simulink model "battery_cell_model"  (R2022b)
settings: Solver=VariableStepAuto  StartTime=0.0  StopTime=t_final  MaxStep=0.1  RelTol=1e-3
values from neighbouring files (symbols this model uses):
  Battery_Model = 6    [OB_N_2_udds.mat]    (also in OB_N_3_(2).mat; OB_N_3_fs.mat = 5; OB_N_3_udds.mat; OB_N_4_udds.mat)
  c =     [OB_N_2_udds.mat]    (also in OB_N_3_(2).mat; OB_N_3_fs.mat; OB_N_3_udds.mat; OB_N_4_udds.mat)
  initial_n = [0.0224016218596 0.0224016218596 0.0224016218596 0.0224016218596 0.0224016218596 0.0224016218596 0.0224016218596 0.0224016218596 0.0224016218596 0.0224016218596 0.0224016218596 0.0224016218596 ... (32 elements, 1x32)]    [OB_N_2_udds.mat]    (also in OB_N_3_(2).mat = [0.0124453454776 0.0124453454776 0.0124453454776 0.012445345; OB_N_3_fs.mat = [0.0248906909552 0.0248906909552 0.0248906909552 0.024890690; OB_N_3_udds.mat; OB_N_4_udds.mat)
  initial_n_lm = [0.0224016218596 0.0224016218596 0.0224016218596 0.0224016218596 0.0224016218596 0.0224016218596 0.0224016218596 0.0224016218596 0.0224016218596 0.0224016218596 0.0224016218596 0.0224016218596 ... (49 elements, 1x49)]    [OB_N_2_udds.mat]    (also in OB_N_3_(2).mat = [0.0124453454776 0.0124453454776 0.0124453454776 0.012445345; OB_N_3_fs.mat = [0.0248906909552 0.0248906909552 0.0248906909552 0.024890690; OB_N_3_udds.mat; OB_N_4_udds.mat)
  initial_n_nm = [0.0224016218596 0.0224016218596 0.0224016218596 0.0224016218596 0.0224016218596 0.0224016218596 0.0224016218596 0.0224016218596 0.0224016218596 0.0224016218596 0.0224016218596 0.0224016218596 ... (49 elements, 1x49)]    [OB_N_2_udds.mat]    (also in OB_N_3_(2).mat = [0.0124453454776 0.0124453454776 0.0124453454776 0.012445345; OB_N_3_fs.mat = [0.0248906909552 0.0248906909552 0.0248906909552 0.024890690; OB_N_3_udds.mat; OB_N_4_udds.mat)
  initial_p = [0.002349018 0.002349018 0.002349018 0.002349018 0.002349018 0.002349018 0.002349018 0.002349018 0.002349018 0.002349018 0.002349018 0.002349018 ... (32 elements, 1x32)]    [OB_N_2_udds.mat]    (also in OB_N_3_(2).mat = [0.00900837 0.00900837 0.00900837 0.00900837 0.00900837 0.00; OB_N_3_fs.mat = [0.00068418 0.00068418 0.00068418 0.00068418 0.00068418 0.00; OB_N_3_udds.mat; OB_N_4_udds.mat)
  initial_p_lm = [0.002349018 0.002349018 0.002349018 0.002349018 0.002349018 0.002349018 0.002349018 0.002349018 0.002349018 0.002349018 0.002349018 0.002349018 ... (49 elements, 1x49)]    [OB_N_2_udds.mat]    (also in OB_N_3_(2).mat = [0.00900837 0.00900837 0.00900837 0.00900837 0.00900837 0.00; OB_N_3_fs.mat = [0.00068418 0.00068418 0.00068418 0.00068418 0.00068418 0.00; OB_N_3_udds.mat; OB_N_4_udds.mat)
  initial_p_nm = [0.002349018 0.002349018 0.002349018 0.002349018 0.002349018 0.002349018 0.002349018 0.002349018 0.002349018 0.002349018 0.002349018 0.002349018 ... (49 elements, 1x49)]    [OB_N_2_udds.mat]    (also in OB_N_3_(2).mat = [0.00900837 0.00900837 0.00900837 0.00900837 0.00900837 0.00; OB_N_3_fs.mat = [0.00068418 0.00068418 0.00068418 0.00068418 0.00068418 0.00; OB_N_3_udds.mat; OB_N_4_udds.mat)
  x_initial_n = [0.0224016218596 0]    [OB_N_2_udds.mat]    (also in OB_N_3_(2).mat = [0.0124453454776 0 0]; OB_N_3_fs.mat = [0.0248906909552 0 0]; OB_N_3_udds.mat = [0.0224016218596 0 0]; OB_N_4_udds.mat = [0.0224016218596 0 0 0])
  x_initial_n_pade = [-7348.24708226 0 0 0 0 0]    [OB_N_2_udds.mat]    (also in OB_N_3_(2).mat = [-4082.35949015 0 0 0 0 0]; OB_N_3_fs.mat = [-8164.71898029 0 0 0 0 0]; OB_N_3_udds.mat; OB_N_4_udds.mat)
  x_initial_n_pade_D = [-2.366529513 0 0 0]    [OB_N_2_udds.mat]    (also in OB_N_3_(2).mat = [-1.31473861834 0 0 0]; OB_N_3_fs.mat = [-0.000240313391395 0 0]; OB_N_3_udds.mat; OB_N_4_udds.mat)
  x_initial_p = [0.002349018 0]    [OB_N_2_udds.mat]    (also in OB_N_3_(2).mat = [0.00900837 0 0]; OB_N_3_fs.mat = [0.00068418 0 0]; OB_N_3_udds.mat = [0.002349018 0 0]; OB_N_4_udds.mat = [0.002349018 0 0 0])
  x_initial_p_pade = [1152.00829448 0 0 0 0 0]    [OB_N_2_udds.mat]    (also in OB_N_3_(2).mat = [4417.8958866 0 0 0 0 0]; OB_N_3_fs.mat = [335.53639645 0 0 0 0 0]; OB_N_3_udds.mat; OB_N_4_udds.mat)
  x_initial_p_pade_D = [1152.00829448 0 0 0]    [OB_N_2_udds.mat]    (also in OB_N_3_(2).mat = [4417.8958866 0 0 0]; OB_N_3_fs.mat = [335.53639645 0 0]; OB_N_3_udds.mat; OB_N_4_udds.mat)
settings Model: Creator=moonjihoon  LastModifiedBy=moonjihoon
settings SolverCC: AlgebraicLoopSolver=TrustRegion
settings DebuggingCC: UnconnectedInputMsg=warning  UnconnectedOutputMsg=warning  UnconnectedLineMsg=warning  SFMachineParentedDataDiag=warning
settings ModelReferenceCC: EnableRefExpFcnMdlSchedulingChecks=on
settings RTWCC: DLArmComputeVersion=19.05

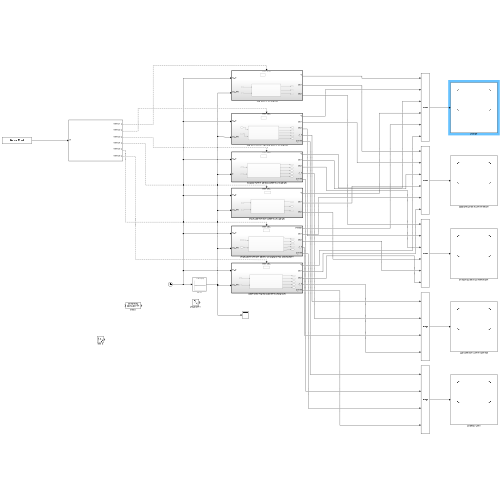
[thumbnail: Simulink's stored preview of the top-level diagram]
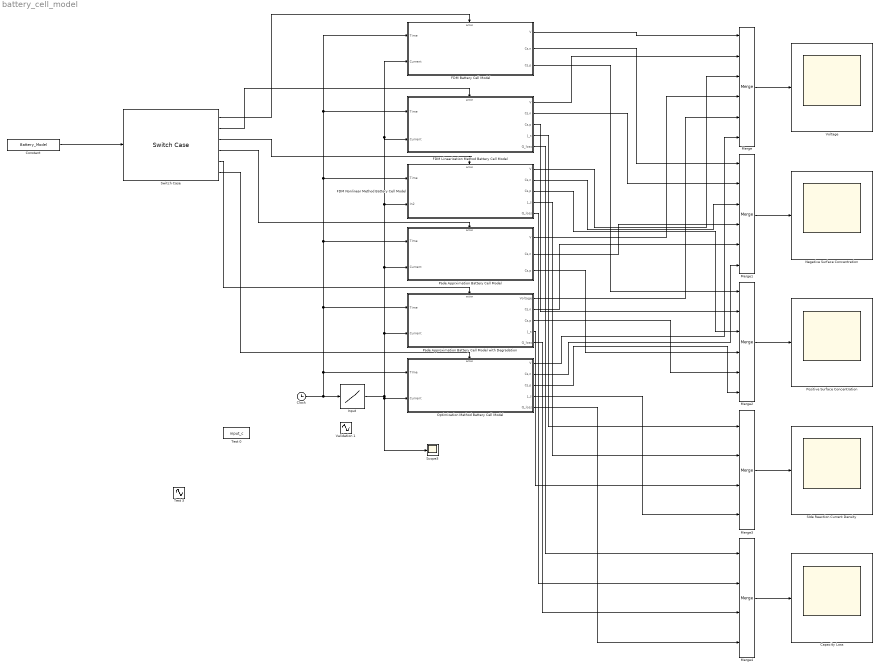
== system battery_cell_model ==
  Capacity Loss : Scope
  Clock : Clock
  Constant : Constant  Value=Battery_Model
  FDM Battery Cell Model : Subsystem  TreatAsAtomicUnit=on
  FDM Linearization Method Battery Cell Model : Subsystem  TreatAsAtomicUnit=on
  FDM Nonlinear Method Battery Cell Model : Subsystem  TreatAsAtomicUnit=on
  Input : Lookup_n-D  NumberOfTableDimensions=1  BreakpointsForDimension1=t  Table=u  InternalRulePriority=Speed  RndMeth=Simplest
  Merge : Merge  Inputs=6
  Merge1 : Merge  Inputs=6
  Merge2 : Merge  Inputs=6
  Merge3 : Merge  Inputs=4
  Merge4 : Merge  Inputs=4
  Negative Surface Concentration : Scope
  Optimization Method Battery Cell Model : Subsystem  TreatAsAtomicUnit=on
  Pade Approximation Battery Cell Model with Degradation : Subsystem  TreatAsAtomicUnit=on
  Pade Apprximation Battery Cell Model : Subsystem  TreatAsAtomicUnit=on
  Positive Surface Concentration : Scope
  SIde Reaction Current Density : Scope
  Scope3 : Scope
  Switch Case : SwitchCase  CaseConditions={1,2,3,4,5,6}  ShowDefaultCase=off
  Test 0 : MATLABFcn  MATLABFcn=input_c
  Test 3 : Sin  Amplitude=6  Frequency=0.03  Phase=3*pi/2  SampleTime=0
  Validation 1 : Sin  Amplitude=5  Frequency=0.02  SampleTime=0
  Voltage : Scope
  wires:
  Optimization Method Battery Cell Model/1(V) -> Merge/6
  Optimization Method Battery Cell Model/2(Cs,n) -> Merge1/6
  Optimization Method Battery Cell Model/3(Cs,p) -> Merge2/6
  FDM Battery Cell Model/2(Cs,n) -> Merge1/1
  FDM Battery Cell Model/3(Cs,p) -> Merge2/1
  FDM Battery Cell Model/1(V) -> Merge/1
  FDM Linearization Method Battery Cell Model/1(V) -> Merge/2
  FDM Linearization Method Battery Cell Model/2(Cs,n) -> Merge1/2
  FDM Linearization Method Battery Cell Model/3(Cs,p) -> Merge2/2
  FDM Linearization Method Battery Cell Model/4(J_s) -> Merge3/1
  FDM Nonlinear Method Battery Cell Model/1(V) -> Merge/3
  FDM Nonlinear Method Battery Cell Model/2(Cs,n) -> Merge1/3
  FDM Nonlinear Method Battery Cell Model/3(Cs,p) -> Merge2/3
  FDM Nonlinear Method Battery Cell Model/4(J_s) -> Merge3/2
  Pade Apprximation Battery Cell Model/1(V) -> Merge/4
  Pade Approximation Battery Cell Model with Degradation/3(Cs,p) -> Merge2/5
  Pade Approximation Battery Cell Model with Degradation/1(Voltage) -> Merge/5
  Pade Approximation Battery Cell Model with Degradation/2(Cs,n) -> Merge1/5
  Switch Case/1 -> FDM Battery Cell Model/Action
  Switch Case/2 -> FDM Linearization Method Battery Cell Model/Action
  Switch Case/3 -> FDM Nonlinear Method Battery Cell Model/Action
  Pade Apprximation Battery Cell Model/3(Cs,p) -> Merge2/4
  Pade Apprximation Battery Cell Model/2(Cs,n) -> Merge1/4
  Constant/1 -> Switch Case/1
  Switch Case/4 -> Pade Apprximation Battery Cell Model/Action
  Switch Case/5 -> Pade Approximation Battery Cell Model with Degradation/Action
  Switch Case/6 -> Optimization Method Battery Cell Model/Action
  Merge/1 -> Voltage/1
  Merge1/1 -> Negative Surface Concentration/1
  Merge2/1 -> Positive Surface Concentration/1
  Merge3/1 -> SIde Reaction Current Density/1
  FDM Linearization Method Battery Cell Model/5(Q_loss) -> Merge4/1
  Merge4/1 -> Capacity Loss/1
  FDM Nonlinear Method Battery Cell Model/5(Q_loss) -> Merge4/2
  Pade Approximation Battery Cell Model with Degradation/4(J_s) -> Merge3/3
  Pade Approximation Battery Cell Model with Degradation/5(Q_loss) -> Merge4/3
  Input/1 -> Optimization Method Battery Cell Model/2(Current), Scope3/1, Pade Apprximation Battery Cell Model/2(Current), FDM Nonlinear Method Battery Cell Model/2(In2), FDM Battery Cell Model/2(Current), FDM Linearization Method Battery Cell Model/2(Current), Pade Approximation Battery Cell Model with Degradation/2(Current)
  Clock/1 -> Input/1, Pade Apprximation Battery Cell Model/1(TIme), FDM Nonlinear Method Battery Cell Model/1(Time), FDM Battery Cell Model/1(Time), FDM Linearization Method Battery Cell Model/1(Time), Pade Approximation Battery Cell Model with Degradation/1(Time), Optimization Method Battery Cell Model/1(TIme)
  Optimization Method Battery Cell Model/4(J_s) -> Merge3/4
  Optimization Method Battery Cell Model/5(Q_loss) -> Merge4/4

== system battery_cell_model/FDM Battery Cell Model ==
  Time : Inport
  Current : Inport  Port=2
  Action Port : ActionPort  ActionPortLabel=case [ 1 ]:
  FDM Battery Cell Model : Subsystem
  V : Outport
  Cs,n : Outport  Port=2
  Cs,p : Outport  Port=3
  wires:
  Time/1 -> FDM Battery Cell Model/1(Time)
  Current/1 -> FDM Battery Cell Model/2(Current)
  FDM Battery Cell Model/1(V) -> V/1
  FDM Battery Cell Model/2(Cs,n) -> Cs,n/1
  FDM Battery Cell Model/3(Cs,p) -> Cs,p/1

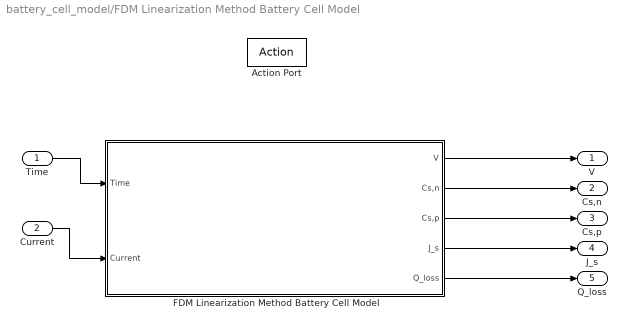
== system battery_cell_model/FDM Linearization Method Battery Cell Model ==
  Time : Inport
  Current : Inport  Port=2
  Action Port : ActionPort  ActionPortLabel=case [ 2 ]:
  FDM Linearization Method Battery Cell Model : Subsystem
  V : Outport
  Cs,n : Outport  Port=2
  Cs,p : Outport  Port=3
  J_s : Outport  Port=4
  Q_loss : Outport  Port=5
  wires:
  Time/1 -> FDM Linearization Method Battery Cell Model/1(Time)
  FDM Linearization Method Battery Cell Model/4(J_s) -> J_s/1
  Current/1 -> FDM Linearization Method Battery Cell Model/2(Current)
  FDM Linearization Method Battery Cell Model/1(V) -> V/1
  FDM Linearization Method Battery Cell Model/2(Cs,n) -> Cs,n/1
  FDM Linearization Method Battery Cell Model/3(Cs,p) -> Cs,p/1
  FDM Linearization Method Battery Cell Model/5(Q_loss) -> Q_loss/1

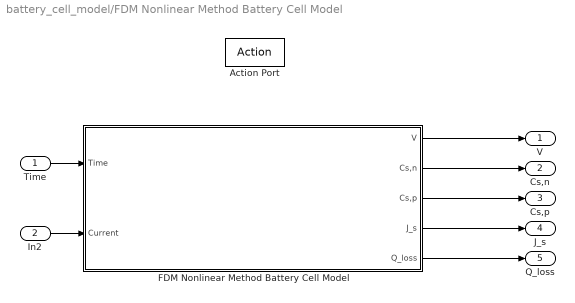
== system battery_cell_model/FDM Nonlinear Method Battery Cell Model ==
  Time : Inport
  In2 : Inport  Port=2
  Action Port : ActionPort  ActionPortLabel=case [ 3 ]:
  FDM Nonlinear Method Battery Cell Model : Subsystem
  V : Outport
  Cs,n : Outport  Port=2
  Cs,p : Outport  Port=3
  J_s : Outport  Port=4
  Q_loss : Outport  Port=5
  wires:
  In2/1 -> FDM Nonlinear Method Battery Cell Model/2(Current)
  Time/1 -> FDM Nonlinear Method Battery Cell Model/1(Time)
  FDM Nonlinear Method Battery Cell Model/1(V) -> V/1
  FDM Nonlinear Method Battery Cell Model/2(Cs,n) -> Cs,n/1
  FDM Nonlinear Method Battery Cell Model/3(Cs,p) -> Cs,p/1
  FDM Nonlinear Method Battery Cell Model/4(J_s) -> J_s/1
  FDM Nonlinear Method Battery Cell Model/5(Q_loss) -> Q_loss/1

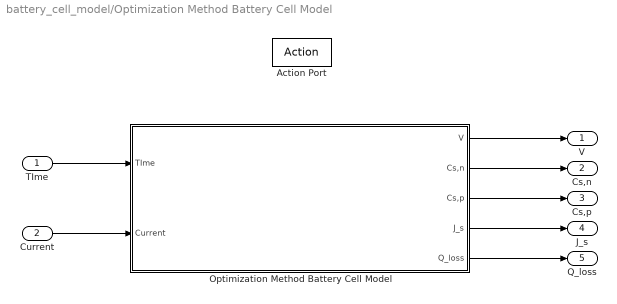
== system battery_cell_model/Optimization Method Battery Cell Model ==
  TIme : Inport
  Current : Inport  Port=2
  Action Port : ActionPort  ActionPortLabel=case [ 6 ]:
  Optimization Method Battery Cell Model : Subsystem
  V : Outport
  Cs,n : Outport  Port=2
  Cs,p : Outport  Port=3
  J_s : Outport  Port=4
  Q_loss : Outport  Port=5
  wires:
  Current/1 -> Optimization Method Battery Cell Model/2(Current)
  TIme/1 -> Optimization Method Battery Cell Model/1(TIme)
  Optimization Method Battery Cell Model/1(V) -> V/1
  Optimization Method Battery Cell Model/2(Cs,n) -> Cs,n/1
  Optimization Method Battery Cell Model/3(Cs,p) -> Cs,p/1
  Optimization Method Battery Cell Model/5(Q_loss) -> Q_loss/1
  Optimization Method Battery Cell Model/4(J_s) -> J_s/1

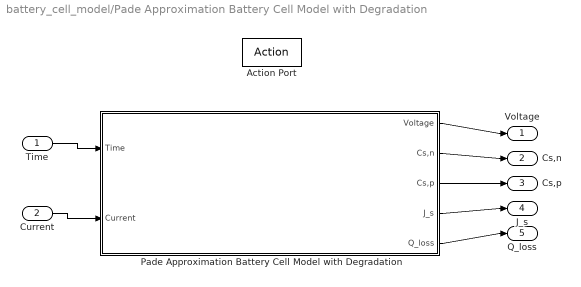
== system battery_cell_model/Pade Approximation Battery Cell Model with Degradation ==
  Time : Inport
  Current : Inport  Port=2
  Action Port : ActionPort  ActionPortLabel=case [ 5 ]:
  Pade Approximation Battery Cell Model with Degradation : Subsystem
  Voltage : Outport
  Cs,n : Outport  Port=2
  Cs,p : Outport  Port=3
  J_s : Outport  Port=4
  Q_loss : Outport  Port=5
  wires:
  Current/1 -> Pade Approximation Battery Cell Model with Degradation/2(Current)
  Time/1 -> Pade Approximation Battery Cell Model with Degradation/1(Time)
  Pade Approximation Battery Cell Model with Degradation/3(Cs,p) -> Cs,p/1
  Pade Approximation Battery Cell Model with Degradation/2(Cs,n) -> Cs,n/1
  Pade Approximation Battery Cell Model with Degradation/1(Voltage) -> Voltage/1
  Pade Approximation Battery Cell Model with Degradation/4(J_s) -> J_s/1
  Pade Approximation Battery Cell Model with Degradation/5(Q_loss) -> Q_loss/1

== system battery_cell_model/Pade Apprximation Battery Cell Model ==
  TIme : Inport
  Current : Inport  Port=2
  Action Port : ActionPort  ActionPortLabel=case [ 4 ]:
  Pade Apprximation Battery Cell Model : Subsystem
  V : Outport
  Cs,n : Outport  Port=2
  Cs,p : Outport  Port=3
  wires:
  Pade Apprximation Battery Cell Model/1(V) -> V/1
  Pade Apprximation Battery Cell Model/2(Cs,n) -> Cs,n/1
  Pade Apprximation Battery Cell Model/3(Cs,p) -> Cs,p/1
  Current/1 -> Pade Apprximation Battery Cell Model/2(Current)
  TIme/1 -> Pade Apprximation Battery Cell Model/1(TIme)

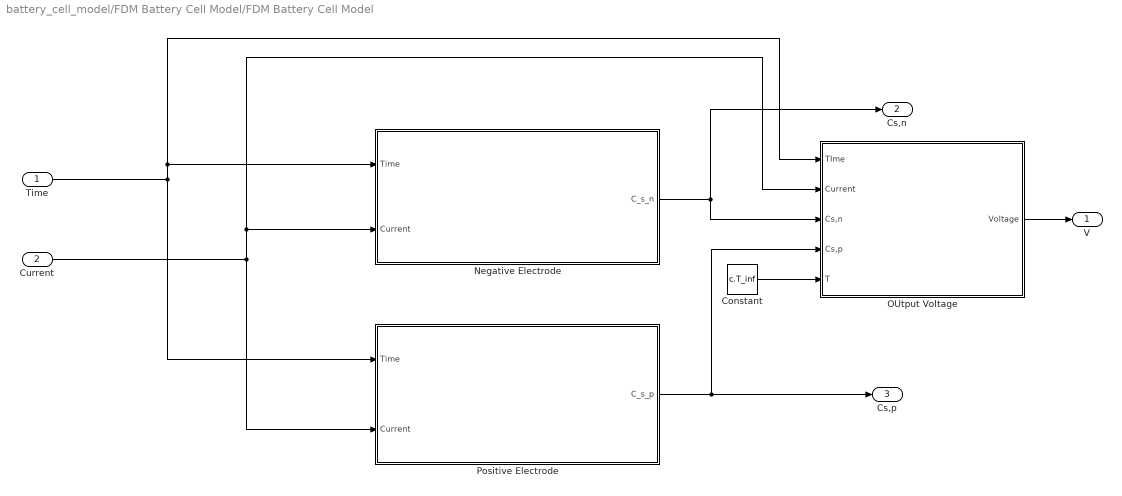
== system battery_cell_model/FDM Battery Cell Model/FDM Battery Cell Model ==
  Time : Inport
  Current : Inport  Port=2
  Constant : Constant  Value=c.T_inf
  Negative Electrode : Subsystem
  OUtput Voltage : Subsystem
  Positive Electrode : Subsystem
  V : Outport
  Cs,n : Outport  Port=2
  Cs,p : Outport  Port=3
  wires:
  Time/1 -> Negative Electrode/1(Time), OUtput Voltage/1(TIme), Positive Electrode/1(Time)
  Current/1 -> OUtput Voltage/2(Current), Negative Electrode/2(Current), Positive Electrode/2(Current)
  Constant/1 -> OUtput Voltage/5(T)
  OUtput Voltage/1(Voltage) -> V/1
  Negative Electrode/1(C_s_n) -> Cs,n/1, OUtput Voltage/3(Cs,n)
  Positive Electrode/1(C_s_p) -> OUtput Voltage/4(Cs,p), Cs,p/1

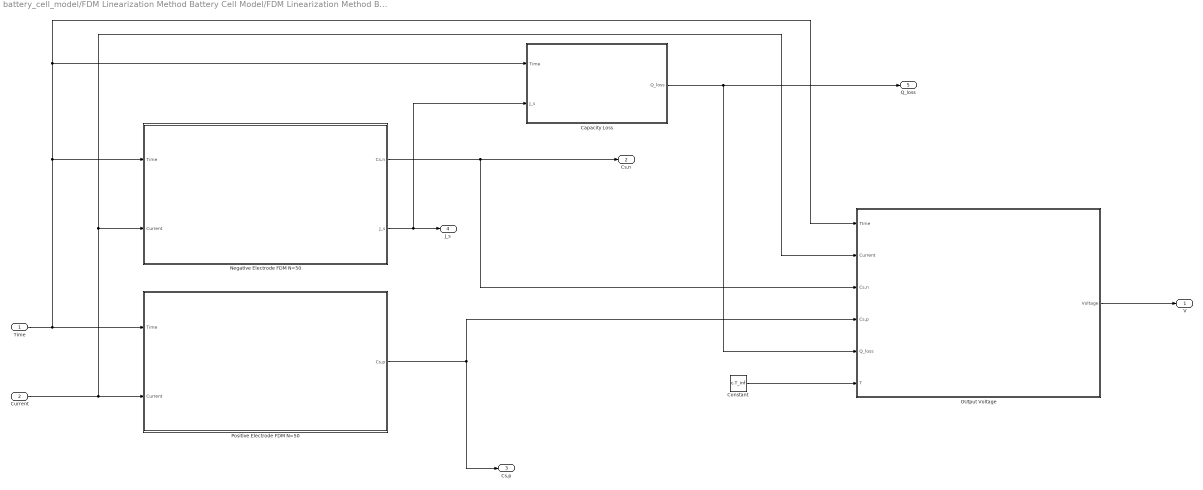
== system battery_cell_model/FDM Linearization Method Battery Cell Model/FDM Linearization Method Battery Cell Model ==
  Time : Inport
  Current : Inport  Port=2
  Capacity Loss : Subsystem
  Constant : Constant  Value=c.T_inf
  Negative Electrode FDM N=50 : Subsystem
  OUtput Voltage : Subsystem
  Positive Electrode FDM N=50 : Subsystem
  V : Outport
  Cs,n : Outport  Port=2
  Cs,p : Outport  Port=3
  J_s : Outport  Port=4
  Q_loss : Outport  Port=5
  wires:
  Constant/1 -> OUtput Voltage/6(T)
  Positive Electrode FDM N=50/1(Cs,p) -> Cs,p/1, OUtput Voltage/4(Cs,p)
  OUtput Voltage/1(Voltage) -> V/1
  Current/1 -> Negative Electrode FDM N=50/2(Current), OUtput Voltage/2(Current), Positive Electrode FDM N=50/2(Current)
  Negative Electrode FDM N=50/2(J_s) -> Capacity Loss/2(J_s), J_s/1
  Negative Electrode FDM N=50/1(Cs,n) -> OUtput Voltage/3(Cs,n), Cs,n/1
  Time/1 -> Capacity Loss/1(Time), OUtput Voltage/1(TIme), Negative Electrode FDM N=50/1(Time), Positive Electrode FDM N=50/1(Time)
  Capacity Loss/1(Q_loss) -> Q_loss/1, OUtput Voltage/5(Q_loss)

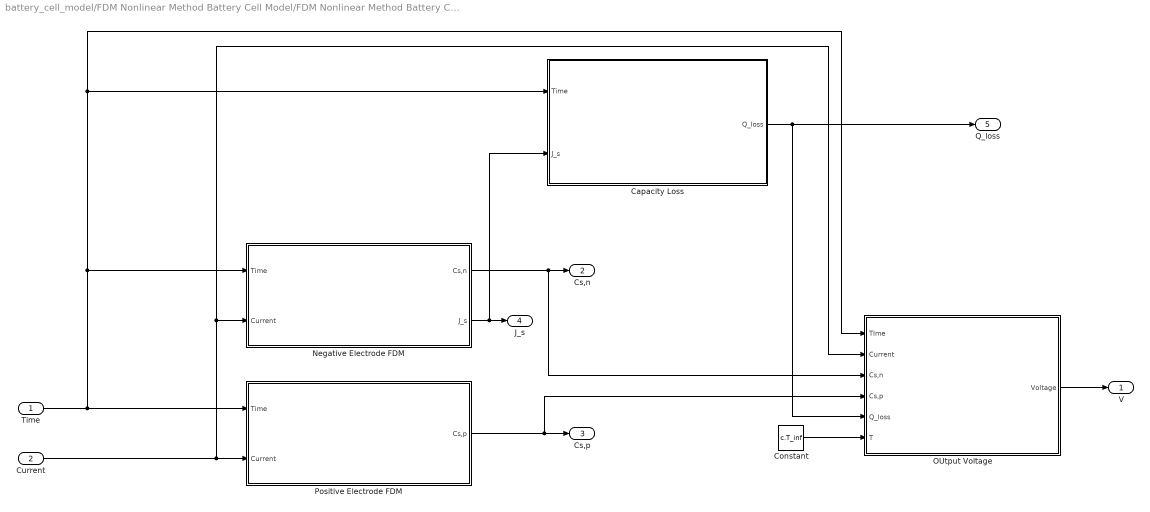
== system battery_cell_model/FDM Nonlinear Method Battery Cell Model/FDM Nonlinear Method Battery Cell Model ==
  Time : Inport
  Current : Inport  Port=2
  Capacity Loss : Subsystem
  Constant : Constant  Value=c.T_inf
  Negative Electrode FDM : Subsystem
  OUtput Voltage : Subsystem
  Positive Electrode FDM : Subsystem
  V : Outport
  Cs,n : Outport  Port=2
  Cs,p : Outport  Port=3
  J_s : Outport  Port=4
  Q_loss : Outport  Port=5
  wires:
  Negative Electrode FDM/2(J_s) -> Capacity Loss/2(J_s), J_s/1
  OUtput Voltage/1(Voltage) -> V/1
  Time/1 -> Negative Electrode FDM/1(Time), Capacity Loss/1(Time), OUtput Voltage/1(TIme), Positive Electrode FDM/1(Time)
  Positive Electrode FDM/1(Cs,p) -> OUtput Voltage/4(Cs,p), Cs,p/1
  Current/1 -> Negative Electrode FDM/2(Current), OUtput Voltage/2(Current), Positive Electrode FDM/2(Current)
  Constant/1 -> OUtput Voltage/6(T)
  Negative Electrode FDM/1(Cs,n) -> OUtput Voltage/3(Cs,n), Cs,n/1
  Capacity Loss/1(Q_loss) -> Q_loss/1, OUtput Voltage/5(Q_loss)

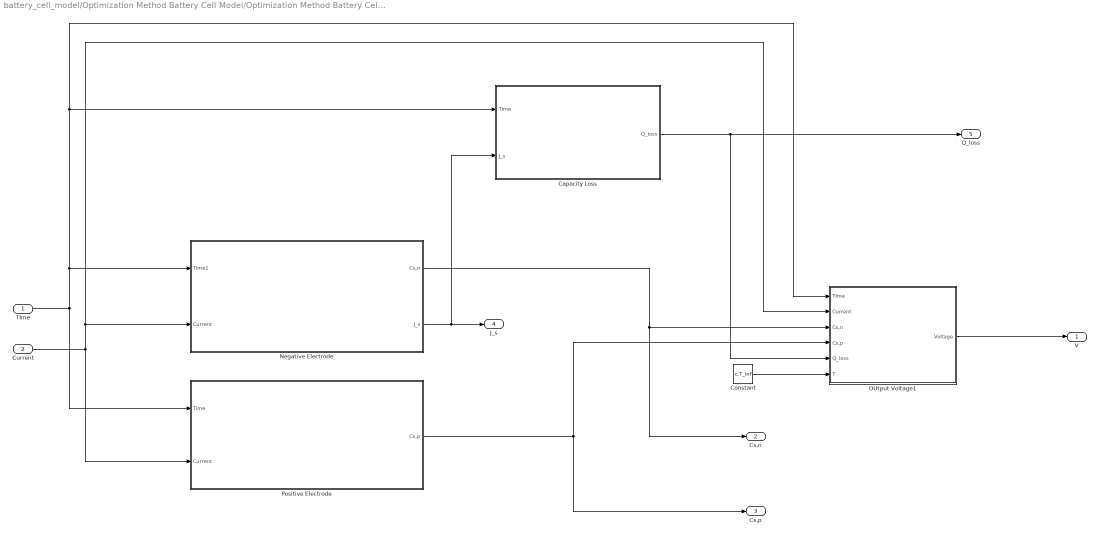
== system battery_cell_model/Optimization Method Battery Cell Model/Optimization Method Battery Cell Model ==
  TIme : Inport
  Current : Inport  Port=2
  Capacity Loss : Subsystem
  Constant : Constant  Value=c.T_inf
  Negative Electrode : Subsystem
  OUtput Voltage1 : Subsystem
  Positive Electrode : Subsystem
  V : Outport
  Cs,n : Outport  Port=2
  Cs,p : Outport  Port=3
  J_s : Outport  Port=4
  Q_loss : Outport  Port=5
  wires:
  Current/1 -> OUtput Voltage1/2(Current), Negative Electrode/2(Current), Positive Electrode/2(Current)
  TIme/1 -> Positive Electrode/1(Time), Capacity Loss/1(Time), OUtput Voltage1/1(TIme), Negative Electrode/1(Time1)
  OUtput Voltage1/1(Voltage) -> V/1
  Negative Electrode/1(Cs,n) -> Cs,n/1, OUtput Voltage1/3(Cs,n)
  Positive Electrode/1(Cs,p) -> Cs,p/1, OUtput Voltage1/4(Cs,p)
  Negative Electrode/2(J_s) -> Capacity Loss/2(J_s), J_s/1
  Capacity Loss/1(Q_loss) -> OUtput Voltage1/5(Q_loss), Q_loss/1
  Constant/1 -> OUtput Voltage1/6(T)

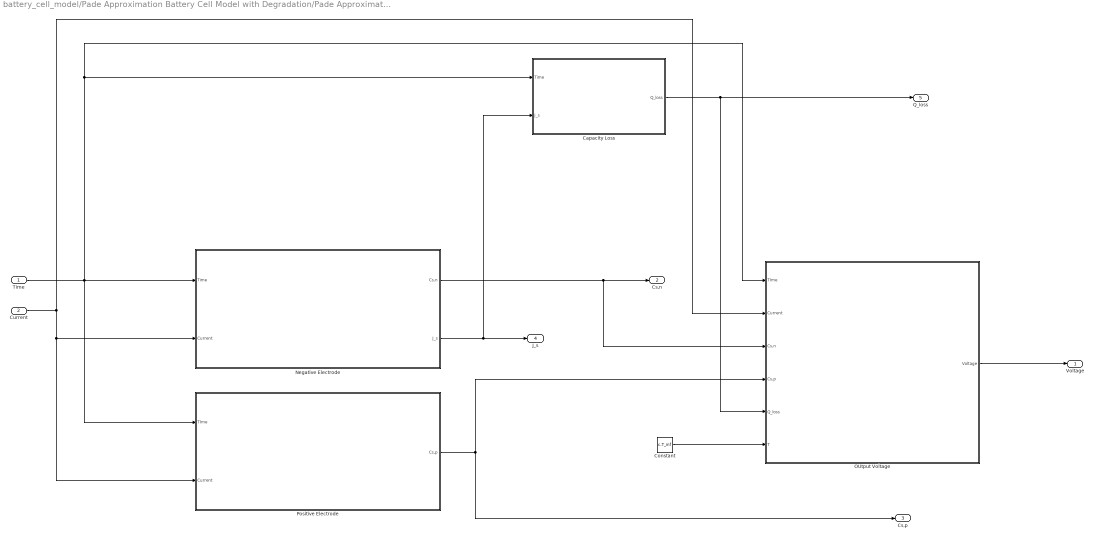
== system battery_cell_model/Pade Approximation Battery Cell Model with Degradation/Pade Approximation Battery Cell Model with Degradation ==
  Time : Inport
  Current : Inport  Port=2
  Capacity Loss : Subsystem
  Constant : Constant  Value=c.T_inf
  Negative Electrode : Subsystem
  OUtput Voltage : Subsystem
  Positive Electrode : Subsystem
  Voltage : Outport
  Cs,n : Outport  Port=2
  Cs,p : Outport  Port=3
  J_s : Outport  Port=4
  Q_loss : Outport  Port=5
  wires:
  Time/1 -> Positive Electrode/1(TIme), Negative Electrode/1(Time), Capacity Loss/1(Time), OUtput Voltage/1(TIme)
  Current/1 -> Positive Electrode/2(Current), Negative Electrode/2(Current), OUtput Voltage/2(Current)
  OUtput Voltage/1(Voltage) -> Voltage/1
  Negative Electrode/1(Cs,n) -> OUtput Voltage/3(Cs,n), Cs,n/1
  Positive Electrode/1(Cs,p) -> Cs,p/1, OUtput Voltage/4(Cs,p)
  Negative Electrode/2(J_s) -> Capacity Loss/2(J_s), J_s/1
  Capacity Loss/1(Q_loss) -> Q_loss/1, OUtput Voltage/5(Q_loss)
  Constant/1 -> OUtput Voltage/6(T)

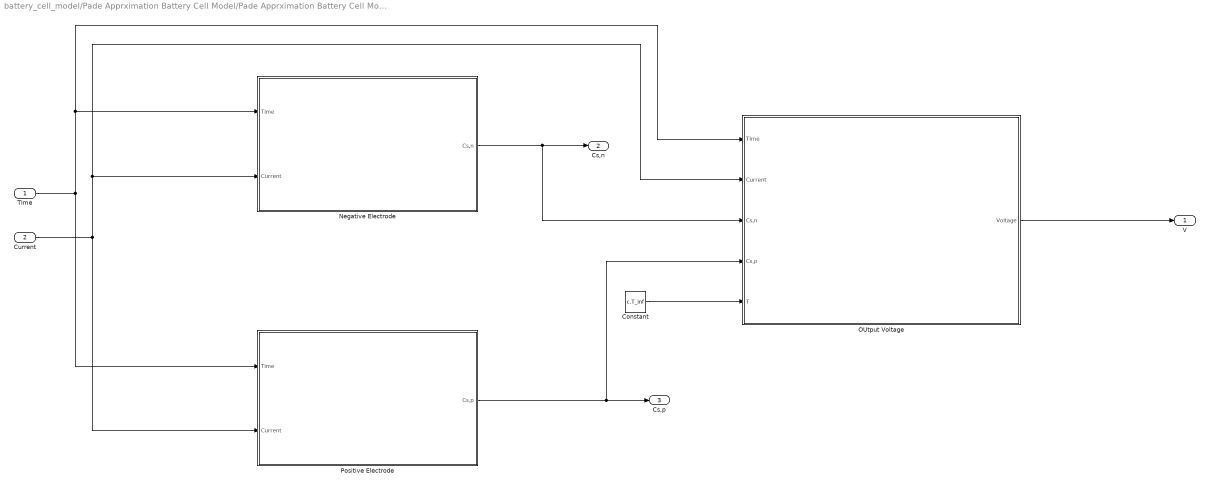
== system battery_cell_model/Pade Apprximation Battery Cell Model/Pade Apprximation Battery Cell Model ==
  TIme : Inport
  Current : Inport  Port=2
  Constant : Constant  Value=c.T_inf
  Negative Electrode : Subsystem
  OUtput Voltage : Subsystem
  Positive Electrode : Subsystem
  V : Outport
  Cs,n : Outport  Port=2
  Cs,p : Outport  Port=3
  wires:
  Current/1 -> OUtput Voltage/2(Current), Negative Electrode/2(Current), Positive Electrode/2(Current)
  TIme/1 -> OUtput Voltage/1(TIme), Negative Electrode/1(Time), Positive Electrode/1(Time)
  OUtput Voltage/1(Voltage) -> V/1
  Constant/1 -> OUtput Voltage/5(T)
  Positive Electrode/1(Cs,p) -> OUtput Voltage/4(Cs,p), Cs,p/1
  Negative Electrode/1(Cs,n) -> OUtput Voltage/3(Cs,n), Cs,n/1

== system battery_cell_model/FDM Battery Cell Model/FDM Battery Cell Model/Negative Electrode ==
  Time : Inport
  Current : Inport  Port=2
  Negative Surface Concentration : Subsystem
  Negative electrode : Subsystem
  C_s_n : Outport
  wires:
  Current/1 -> Negative Surface Concentration/2(Current), Negative electrode/2(In2)
  Negative Surface Concentration/1(C_s_n) -> C_s_n/1
  Time/1 -> Negative Surface Concentration/1(Time), Negative electrode/1(In1)
  Negative electrode/1(Cn) -> Negative Surface Concentration/3(Cn)

== system battery_cell_model/FDM Battery Cell Model/FDM Battery Cell Model/OUtput Voltage ==
  TIme : Inport
  Current : Inport  Port=2
  Cs,n : Inport  Port=3
  Cs,p : Inport  Port=4
  T : Inport  Port=5
  Interpreted MATLAB Function : MATLABFcn  MATLABFcn=output_V
  Mux : Mux  Inputs=5
  Voltage : Outport
  wires:
  TIme/1 -> Mux/1
  Interpreted MATLAB Function/1 -> Voltage/1
  Mux/1 -> Interpreted MATLAB Function/1
  Current/1 -> Mux/2
  Cs,n/1 -> Mux/3
  T/1 -> Mux/5
  Cs,p/1 -> Mux/4

== system battery_cell_model/FDM Battery Cell Model/FDM Battery Cell Model/Positive Electrode ==
  Time : Inport
  Current : Inport  Port=2
  Positive Surface Concentration : Subsystem
  Positive electrode : Subsystem
  C_s_p : Outport
  wires:
  Current/1 -> Positive Surface Concentration/2(Current), Positive electrode/2(Current)
  Time/1 -> Positive Surface Concentration/1(Time), Positive electrode/1(Time)
  Positive Surface Concentration/1(C_s_p) -> C_s_p/1
  Positive electrode/1(Cp) -> Positive Surface Concentration/3(Cp)

== system battery_cell_model/FDM Linearization Method Battery Cell Model/FDM Linearization Method Battery Cell Model/Capacity Loss ==
  Time : Inport
  J_s : Inport  Port=2
  Integrator : Integrator
  Interpreted MATLAB Function : MATLABFcn  MATLABFcn=Capacity_Loss
  Mux : Mux  Inputs=3
  Q_loss : Outport
  wires:
  Mux/1 -> Interpreted MATLAB Function/1
  Time/1 -> Mux/1
  Interpreted MATLAB Function/1 -> Integrator/1
  J_s/1 -> Mux/2
  Integrator/1 -> Mux/3, Q_loss/1

== system battery_cell_model/FDM Linearization Method Battery Cell Model/FDM Linearization Method Battery Cell Model/Negative Electrode FDM N=50 ==
  Time : Inport
  Current : Inport  Port=2
  Negative electrode : Subsystem
  Side reaction current density : Subsystem
  Surface Concentration : Subsystem
  Cs,n : Outport
  J_s : Outport  Port=2
  wires:
  Negative electrode/1(Cs,n) -> Surface Concentration/3(Cs,n)
  Side reaction current density/1(J_s) -> J_s/1
  Time/1 -> Surface Concentration/1(Time), Side reaction current density/1(Time), Negative electrode/1(time)
  Surface Concentration/1(C_s) -> Side reaction current density/3(Cs,n), Cs,n/1
  Current/1 -> Surface Concentration/2(Current), Side reaction current density/2(Current), Negative electrode/2(current)

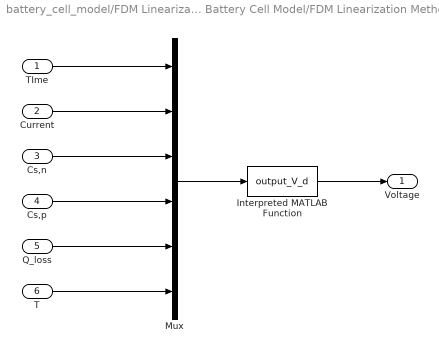
== system battery_cell_model/FDM Linearization Method Battery Cell Model/FDM Linearization Method Battery Cell Model/OUtput Voltage ==
  TIme : Inport
  Current : Inport  Port=2
  Cs,n : Inport  Port=3
  Cs,p : Inport  Port=4
  Q_loss : Inport  Port=5
  T : Inport  Port=6
  Interpreted MATLAB Function : MATLABFcn  MATLABFcn=output_V_d
  Mux : Mux  Inputs=6
  Voltage : Outport
  wires:
  TIme/1 -> Mux/1
  Interpreted MATLAB Function/1 -> Voltage/1
  Mux/1 -> Interpreted MATLAB Function/1
  Current/1 -> Mux/2
  Cs,n/1 -> Mux/3
  T/1 -> Mux/6
  Cs,p/1 -> Mux/4
  Q_loss/1 -> Mux/5

== system battery_cell_model/FDM Linearization Method Battery Cell Model/FDM Linearization Method Battery Cell Model/Positive Electrode FDM N=50 ==
  Time : Inport
  Current : Inport  Port=2
  Positivee electrode : Subsystem
  Surface Concentration : Subsystem
  Cs,p : Outport
  wires:
  Surface Concentration/1(C_s) -> Cs,p/1
  Time/1 -> Surface Concentration/1(Time), Positivee electrode/1(Time)
  Current/1 -> Surface Concentration/2(Current), Positivee electrode/2(Current)
  Positivee electrode/1(Cp) -> Surface Concentration/3(Cp)

== system battery_cell_model/FDM Nonlinear Method Battery Cell Model/FDM Nonlinear Method Battery Cell Model/Capacity Loss ==
  Time : Inport
  J_s : Inport  Port=2
  Integrator : Integrator
  Interpreted MATLAB Function : MATLABFcn  MATLABFcn=Capacity_Loss
  Mux : Mux  Inputs=3
  Q_loss : Outport
  wires:
  Mux/1 -> Interpreted MATLAB Function/1
  Time/1 -> Mux/1
  Interpreted MATLAB Function/1 -> Integrator/1
  J_s/1 -> Mux/2
  Integrator/1 -> Mux/3, Q_loss/1

== system battery_cell_model/FDM Nonlinear Method Battery Cell Model/FDM Nonlinear Method Battery Cell Model/Negative Electrode FDM ==
  Time : Inport
  Current : Inport  Port=2
  Negative Surface Concentration : Subsystem
  Side reaction current density : Subsystem
  State equation : Subsystem
  Cs,n : Outport
  J_s : Outport  Port=2
  wires:
  Side reaction current density/1(J_s) -> J_s/1
  Negative Surface Concentration/1(C_s) -> Cs,n/1, Side reaction current density/3(Cs,n)
  State equation/1(Cn) -> Negative Surface Concentration/3(Cs,n)
  Time/1 -> Negative Surface Concentration/1(Time), Side reaction current density/1(Time), State equation/1(time)
  Current/1 -> Negative Surface Concentration/2(Current), Side reaction current density/2(Current), State equation/2(current)

== system battery_cell_model/FDM Nonlinear Method Battery Cell Model/FDM Nonlinear Method Battery Cell Model/OUtput Voltage ==
  TIme : Inport
  Current : Inport  Port=2
  Cs,n : Inport  Port=3
  Cs,p : Inport  Port=4
  Q_loss : Inport  Port=5
  T : Inport  Port=6
  Interpreted MATLAB Function : MATLABFcn  MATLABFcn=output_V
  Mux : Mux  Inputs=6
  Voltage : Outport
  wires:
  TIme/1 -> Mux/1
  Interpreted MATLAB Function/1 -> Voltage/1
  Mux/1 -> Interpreted MATLAB Function/1
  Current/1 -> Mux/2
  Cs,n/1 -> Mux/3
  T/1 -> Mux/6
  Cs,p/1 -> Mux/4
  Q_loss/1 -> Mux/5

== system battery_cell_model/FDM Nonlinear Method Battery Cell Model/FDM Nonlinear Method Battery Cell Model/Positive Electrode FDM ==
  Time : Inport
  Current : Inport  Port=2
  Positive Surface Concentration : Subsystem
  State equation : Subsystem
  Cs,p : Outport
  wires:
  Positive Surface Concentration/1(C_s) -> Cs,p/1
  Time/1 -> Positive Surface Concentration/1(Time), State equation/1(Time)
  Current/1 -> Positive Surface Concentration/2(Current), State equation/2(Current)
  State equation/1(Cs,p) -> Positive Surface Concentration/3(Cs,p)

== system battery_cell_model/Optimization Method Battery Cell Model/Optimization Method Battery Cell Model/Capacity Loss ==
  Time : Inport
  J_s : Inport  Port=2
  Integrator : Integrator
  Interpreted MATLAB Function : MATLABFcn  MATLABFcn=Capacity_Loss
  Mux : Mux  Inputs=3
  Q_loss : Outport
  wires:
  Mux/1 -> Interpreted MATLAB Function/1
  Time/1 -> Mux/1
  Interpreted MATLAB Function/1 -> Integrator/1
  J_s/1 -> Mux/2
  Integrator/1 -> Mux/3, Q_loss/1

== system battery_cell_model/Optimization Method Battery Cell Model/Optimization Method Battery Cell Model/Negative Electrode ==
  Time1 : Inport
  Current : Inport  Port=2
  Negative Surface concentration : Subsystem
  Negative electrode state equation : Subsystem
  Side reaction current density : Subsystem
  Cs,n : Outport
  J_s : Outport  Port=2
  wires:
  Negative electrode state equation/1(Xn) -> Negative Surface concentration/3(Xn)
  Current/1 -> Side reaction current density/2(Current), Negative Surface concentration/2(u), Negative electrode state equation/2(Current)
  Negative Surface concentration/1(Cs,n) -> Side reaction current density/3(Cs,n), Cs,n/1
  Time1/1 -> Negative electrode state equation/1(Time), Side reaction current density/1(Time), Negative Surface concentration/1(Time)
  Side reaction current density/1(J_s) -> J_s/1

== system battery_cell_model/Optimization Method Battery Cell Model/Optimization Method Battery Cell Model/OUtput Voltage1 ==
  TIme : Inport
  Current : Inport  Port=2
  Cs,n : Inport  Port=3
  Cs,p : Inport  Port=4
  Q_loss : Inport  Port=5
  T : Inport  Port=6
  Interpreted MATLAB Function : MATLABFcn  MATLABFcn=output_V_d
  Mux : Mux  Inputs=6
  Voltage : Outport
  wires:
  TIme/1 -> Mux/1
  Interpreted MATLAB Function/1 -> Voltage/1
  Mux/1 -> Interpreted MATLAB Function/1
  Current/1 -> Mux/2
  Cs,n/1 -> Mux/3
  Q_loss/1 -> Mux/5
  Cs,p/1 -> Mux/4
  T/1 -> Mux/6

== system battery_cell_model/Optimization Method Battery Cell Model/Optimization Method Battery Cell Model/Positive Electrode ==
  Time : Inport
  Current : Inport  Port=2
  Positive Surface concentration : Subsystem
  Positive electrode state equation : Subsystem
  Cs,p : Outport
  wires:
  Positive Surface concentration/1(Cs,p) -> Cs,p/1
  Current/1 -> Positive Surface concentration/2(u), Positive electrode state equation/2(Current)
  Time/1 -> Positive Surface concentration/1(Time), Positive electrode state equation/1(Time)
  Positive electrode state equation/1(Xp) -> Positive Surface concentration/3(Xp)

== system battery_cell_model/Pade Approximation Battery Cell Model with Degradation/Pade Approximation Battery Cell Model with Degradation/Capacity Loss ==
  Time : Inport
  J_s : Inport  Port=2
  Integrator : Integrator
  Interpreted MATLAB Function : MATLABFcn  MATLABFcn=Capacity_Loss
  Mux : Mux  Inputs=3
  Q_loss : Outport
  wires:
  Mux/1 -> Interpreted MATLAB Function/1
  Time/1 -> Mux/1
  Interpreted MATLAB Function/1 -> Integrator/1
  J_s/1 -> Mux/2
  Integrator/1 -> Mux/3, Q_loss/1

== system battery_cell_model/Pade Approximation Battery Cell Model with Degradation/Pade Approximation Battery Cell Model with Degradation/Negative Electrode ==
  Time : Inport
  Current : Inport  Port=2
  Dynamics : Subsystem
  Output C : Subsystem
  Side reaction current density : Subsystem
  Cs,n : Outport
  J_s : Outport  Port=2
  wires:
  Dynamics/1(C_n) -> Output C/3(C_n)
  Current/1 -> Output C/2(Current), Side reaction current density/2(Current), Dynamics/2(Current)
  Side reaction current density/1(J_s) -> J_s/1
  Time/1 -> Side reaction current density/1(Time), Output C/1(Time), Dynamics/1(Time)
  Output C/1(Cs,n) -> Side reaction current density/3(Cs,n), Cs,n/1

== system battery_cell_model/Pade Approximation Battery Cell Model with Degradation/Pade Approximation Battery Cell Model with Degradation/OUtput Voltage ==
  TIme : Inport
  Current : Inport  Port=2
  Cs,n : Inport  Port=3
  Cs,p : Inport  Port=4
  Q_loss : Inport  Port=5
  T : Inport  Port=6
  Interpreted MATLAB Function : MATLABFcn  MATLABFcn=output_V_d
  Mux : Mux  Inputs=6
  Voltage : Outport
  wires:
  TIme/1 -> Mux/1
  Interpreted MATLAB Function/1 -> Voltage/1
  Mux/1 -> Interpreted MATLAB Function/1
  Current/1 -> Mux/2
  Cs,n/1 -> Mux/3
  Cs,p/1 -> Mux/4
  T/1 -> Mux/6
  Q_loss/1 -> Mux/5

== system battery_cell_model/Pade Approximation Battery Cell Model with Degradation/Pade Approximation Battery Cell Model with Degradation/Positive Electrode ==
  TIme : Inport
  Current : Inport  Port=2
  Dynamics : Subsystem
  Output C : Subsystem
  Cs,p : Outport
  wires:
  Current/1 -> Dynamics/2(Current)
  TIme/1 -> Output C/1(Time), Dynamics/1(Time)
  Dynamics/1(C_p) -> Output C/2(C_p)
  Output C/1(Cs,p) -> Cs,p/1

== system battery_cell_model/Pade Apprximation Battery Cell Model/Pade Apprximation Battery Cell Model/Negative Electrode ==
  Time : Inport
  Current : Inport  Port=2
  Dynamics : Subsystem
  Output C : Subsystem
  Cs,n : Outport
  wires:
  Output C/1(Cs,n) -> Cs,n/1
  Time/1 -> Output C/1(Time), Dynamics/1(Time)
  Dynamics/1(C_n) -> Output C/2(C_n)
  Current/1 -> Dynamics/2(Current)

== system battery_cell_model/Pade Apprximation Battery Cell Model/Pade Apprximation Battery Cell Model/OUtput Voltage ==
  TIme : Inport
  Current : Inport  Port=2
  Cs,n : Inport  Port=3
  Cs,p : Inport  Port=4
  T : Inport  Port=5
  Interpreted MATLAB Function : MATLABFcn  MATLABFcn=output_V
  Mux : Mux  Inputs=5
  Voltage : Outport
  wires:
  TIme/1 -> Mux/1
  Interpreted MATLAB Function/1 -> Voltage/1
  Mux/1 -> Interpreted MATLAB Function/1
  Current/1 -> Mux/2
  Cs,n/1 -> Mux/3
  T/1 -> Mux/5
  Cs,p/1 -> Mux/4

== system battery_cell_model/Pade Apprximation Battery Cell Model/Pade Apprximation Battery Cell Model/Positive Electrode ==
  Time : Inport
  Current : Inport  Port=2
  Dynamics : Subsystem
  Output C : Subsystem
  Cs,p : Outport
  wires:
  Output C/1(Cs,p) -> Cs,p/1
  Time/1 -> Output C/1(Time), Dynamics/1(Time)
  Dynamics/1(C_p) -> Output C/2(C_p)
  Current/1 -> Dynamics/2(Current)

== system battery_cell_model/FDM Battery Cell Model/FDM Battery Cell Model/Negative Electrode/Negative Surface Concentration ==
  Time : Inport
  Current : Inport  Port=2
  Cn : Inport  Port=3
  Interpreted MATLAB Function : MATLABFcn  MATLABFcn=output_C_FDM_n
  Mux : Mux  Inputs=3
  C_s_n : Outport
  wires:
  Interpreted MATLAB Function/1 -> C_s_n/1
  Time/1 -> Mux/1
  Current/1 -> Mux/2
  Mux/1 -> Interpreted MATLAB Function/1
  Cn/1 -> Mux/3

== system battery_cell_model/FDM Battery Cell Model/FDM Battery Cell Model/Negative Electrode/Negative electrode ==
  In1 : Inport
  In2 : Inport  Port=2
  Integrator : Integrator  InitialCondition=initial_n
  Interpreted MATLAB Function : MATLABFcn  MATLABFcn=state_eqns_fdm_n
  Mux : Mux  Inputs=3
  Cn : Outport
  wires:
  Interpreted MATLAB Function/1 -> Integrator/1
  In1/1 -> Mux/1
  In2/1 -> Mux/2
  Mux/1 -> Interpreted MATLAB Function/1
  Integrator/1 -> Cn/1, Mux/3

== system battery_cell_model/FDM Battery Cell Model/FDM Battery Cell Model/Positive Electrode/Positive Surface Concentration ==
  Time : Inport
  Current : Inport  Port=2
  Cp : Inport  Port=3
  Interpreted MATLAB Function : MATLABFcn  MATLABFcn=output_C_FDM_p
  Mux : Mux  Inputs=3
  C_s_p : Outport
  wires:
  Interpreted MATLAB Function/1 -> C_s_p/1
  Time/1 -> Mux/1
  Current/1 -> Mux/2
  Mux/1 -> Interpreted MATLAB Function/1
  Cp/1 -> Mux/3

== system battery_cell_model/FDM Battery Cell Model/FDM Battery Cell Model/Positive Electrode/Positive electrode ==
  Time : Inport
  Current : Inport  Port=2
  Integrator : Integrator  InitialCondition=initial_p
  Interpreted MATLAB Function : MATLABFcn  MATLABFcn=state_eqns_fdm_p
  Mux : Mux  Inputs=3
  Cp : Outport
  wires:
  Interpreted MATLAB Function/1 -> Integrator/1
  Time/1 -> Mux/1
  Current/1 -> Mux/2
  Mux/1 -> Interpreted MATLAB Function/1
  Integrator/1 -> Cp/1, Mux/3

== system battery_cell_model/FDM Linearization Method Battery Cell Model/FDM Linearization Method Battery Cell Model/Negative Electrode FDM N=50/Negative electrode ==
  time : Inport
  current : Inport  Port=2
  Integrator : Integrator  InitialCondition=initial_n_lm
  Interpreted MATLAB Function : MATLABFcn  MATLABFcn=state_eqns_fdm_lm_n
  Mux : Mux  Inputs=3
  Cs,n : Outport
  wires:
  Interpreted MATLAB Function/1 -> Integrator/1
  time/1 -> Mux/1
  current/1 -> Mux/2
  Mux/1 -> Interpreted MATLAB Function/1
  Integrator/1 -> Mux/3, Cs,n/1

== system battery_cell_model/FDM Linearization Method Battery Cell Model/FDM Linearization Method Battery Cell Model/Negative Electrode FDM N=50/Side reaction current density ==
  Time : Inport
  Current : Inport  Port=2
  Cs,n : Inport  Port=3
  Interpreted MATLAB Function : MATLABFcn  MATLABFcn=side_reaction
  Mux : Mux  Inputs=3
  J_s : Outport
  wires:
  Interpreted MATLAB Function/1 -> J_s/1
  Time/1 -> Mux/1
  Current/1 -> Mux/2
  Mux/1 -> Interpreted MATLAB Function/1
  Cs,n/1 -> Mux/3

== system battery_cell_model/FDM Linearization Method Battery Cell Model/FDM Linearization Method Battery Cell Model/Negative Electrode FDM N=50/Surface Concentration ==
  Time : Inport
  Current : Inport  Port=2
  Cs,n : Inport  Port=3
  Interpreted MATLAB Function : MATLABFcn  MATLABFcn=output_C_fdm_lm_n
  Mux : Mux  Inputs=3
  C_s : Outport
  wires:
  Interpreted MATLAB Function/1 -> C_s/1
  Cs,n/1 -> Mux/3
  Current/1 -> Mux/2
  Mux/1 -> Interpreted MATLAB Function/1
  Time/1 -> Mux/1

== system battery_cell_model/FDM Linearization Method Battery Cell Model/FDM Linearization Method Battery Cell Model/Positive Electrode FDM N=50/Positivee electrode ==
  Time : Inport
  Current : Inport  Port=2
  Integrator : Integrator  InitialCondition=initial_p_lm
  Interpreted MATLAB Function : MATLABFcn  MATLABFcn=state_eqns_fdm_lm_p
  Mux : Mux  Inputs=3
  Cp : Outport
  wires:
  Interpreted MATLAB Function/1 -> Integrator/1
  Time/1 -> Mux/1
  Current/1 -> Mux/2
  Mux/1 -> Interpreted MATLAB Function/1
  Integrator/1 -> Cp/1, Mux/3

== system battery_cell_model/FDM Linearization Method Battery Cell Model/FDM Linearization Method Battery Cell Model/Positive Electrode FDM N=50/Surface Concentration ==
  Time : Inport
  Current : Inport  Port=2
  Cp : Inport  Port=3
  Interpreted MATLAB Function : MATLABFcn  MATLABFcn=output_C_fdm_lm_p
  Mux : Mux  Inputs=3
  C_s : Outport
  wires:
  Interpreted MATLAB Function/1 -> C_s/1
  Time/1 -> Mux/1
  Current/1 -> Mux/2
  Cp/1 -> Mux/3
  Mux/1 -> Interpreted MATLAB Function/1

== system battery_cell_model/FDM Nonlinear Method Battery Cell Model/FDM Nonlinear Method Battery Cell Model/Negative Electrode FDM/Negative Surface Concentration ==
  Time : Inport
  Current : Inport  Port=2
  Cs,n : Inport  Port=3
  Interpreted MATLAB Function : MATLABFcn  MATLABFcn=output_C_fdm_nm_n
  Mux : Mux  Inputs=3
  C_s : Outport
  wires:
  Interpreted MATLAB Function/1 -> C_s/1
  Cs,n/1 -> Mux/3
  Current/1 -> Mux/2
  Mux/1 -> Interpreted MATLAB Function/1
  Time/1 -> Mux/1

== system battery_cell_model/FDM Nonlinear Method Battery Cell Model/FDM Nonlinear Method Battery Cell Model/Negative Electrode FDM/Side reaction current density ==
  Time : Inport
  Current : Inport  Port=2
  Cs,n : Inport  Port=3
  Interpreted MATLAB Function : MATLABFcn  MATLABFcn=side_reaction_NM
  Mux : Mux  Inputs=3
  J_s : Outport
  wires:
  Interpreted MATLAB Function/1 -> J_s/1
  Time/1 -> Mux/1
  Current/1 -> Mux/2
  Mux/1 -> Interpreted MATLAB Function/1
  Cs,n/1 -> Mux/3

== system battery_cell_model/FDM Nonlinear Method Battery Cell Model/FDM Nonlinear Method Battery Cell Model/Negative Electrode FDM/State equation ==
  time : Inport
  current : Inport  Port=2
  Integrator : Integrator  InitialCondition=initial_n_nm
  Interpreted MATLAB Function : MATLABFcn  MATLABFcn=state_eqns_fdm_nm_n
  Mux : Mux  Inputs=3
  Cn : Outport
  wires:
  Interpreted MATLAB Function/1 -> Integrator/1
  time/1 -> Mux/1
  current/1 -> Mux/2
  Mux/1 -> Interpreted MATLAB Function/1
  Integrator/1 -> Mux/3, Cn/1

== system battery_cell_model/FDM Nonlinear Method Battery Cell Model/FDM Nonlinear Method Battery Cell Model/Positive Electrode FDM/Positive Surface Concentration ==
  Time : Inport
  Current : Inport  Port=2
  Cs,p : Inport  Port=3
  Interpreted MATLAB Function : MATLABFcn  MATLABFcn=output_C_fdm_nm_p
  Mux : Mux  Inputs=3
  C_s : Outport
  wires:
  Interpreted MATLAB Function/1 -> C_s/1
  Time/1 -> Mux/1
  Current/1 -> Mux/2
  Cs,p/1 -> Mux/3
  Mux/1 -> Interpreted MATLAB Function/1

== system battery_cell_model/FDM Nonlinear Method Battery Cell Model/FDM Nonlinear Method Battery Cell Model/Positive Electrode FDM/State equation ==
  Time : Inport
  Current : Inport  Port=2
  Integrator : Integrator  InitialCondition=initial_p_nm
  Interpreted MATLAB Function : MATLABFcn  MATLABFcn=state_eqns_fdm_nm_p
  Mux : Mux  Inputs=3
  Cs,p : Outport
  wires:
  Interpreted MATLAB Function/1 -> Integrator/1
  Time/1 -> Mux/1
  Current/1 -> Mux/2
  Mux/1 -> Interpreted MATLAB Function/1
  Integrator/1 -> Cs,p/1, Mux/3

== system battery_cell_model/Optimization Method Battery Cell Model/Optimization Method Battery Cell Model/Negative Electrode/Negative Surface concentration ==
  Time : Inport
  u : Inport  Port=2
  Xn : Inport  Port=3
  Interpreted MATLAB Function1 : MATLABFcn  MATLABFcn=output_C_OB_n
  Mux : Mux  Inputs=3
  Cs,n : Outport
  wires:
  Time/1 -> Mux/1
  Mux/1 -> Interpreted MATLAB Function1/1
  Interpreted MATLAB Function1/1 -> Cs,n/1
  Xn/1 -> Mux/3
  u/1 -> Mux/2

== system battery_cell_model/Optimization Method Battery Cell Model/Optimization Method Battery Cell Model/Negative Electrode/Negative electrode state equation ==
  Time : Inport
  Current : Inport  Port=2
  Integrator : Integrator  InitialCondition=x_initial_n
  Interpreted MATLAB Function : MATLABFcn  MATLABFcn=state_eqns_n_OB
  Mux : Mux  Inputs=3
  Xn : Outport
  wires:
  Current/1 -> Mux/2
  Time/1 -> Mux/1
  Interpreted MATLAB Function/1 -> Integrator/1
  Mux/1 -> Interpreted MATLAB Function/1
  Integrator/1 -> Xn/1, Mux/3

== system battery_cell_model/Optimization Method Battery Cell Model/Optimization Method Battery Cell Model/Negative Electrode/Side reaction current density ==
  Time : Inport
  Current : Inport  Port=2
  Cs,n : Inport  Port=3
  Interpreted MATLAB Function : MATLABFcn  MATLABFcn=side_reaction
  Mux : Mux  Inputs=3
  J_s : Outport
  wires:
  Interpreted MATLAB Function/1 -> J_s/1
  Time/1 -> Mux/1
  Current/1 -> Mux/2
  Mux/1 -> Interpreted MATLAB Function/1
  Cs,n/1 -> Mux/3

== system battery_cell_model/Optimization Method Battery Cell Model/Optimization Method Battery Cell Model/Positive Electrode/Positive Surface concentration ==
  Time : Inport
  u : Inport  Port=2
  Xp : Inport  Port=3
  Interpreted MATLAB Function1 : MATLABFcn  MATLABFcn=output_C_OB_p
  Mux : Mux  Inputs=3
  Cs,p : Outport
  wires:
  Time/1 -> Mux/1
  Mux/1 -> Interpreted MATLAB Function1/1
  Interpreted MATLAB Function1/1 -> Cs,p/1
  Xp/1 -> Mux/3
  u/1 -> Mux/2

== system battery_cell_model/Optimization Method Battery Cell Model/Optimization Method Battery Cell Model/Positive Electrode/Positive electrode state equation ==
  Time : Inport
  Current : Inport  Port=2
  Integrator : Integrator  InitialCondition=x_initial_p
  Interpreted MATLAB Function : MATLABFcn  MATLABFcn=state_eqns_p_OB
  Mux : Mux  Inputs=3
  Xp : Outport
  wires:
  Current/1 -> Mux/2
  Time/1 -> Mux/1
  Interpreted MATLAB Function/1 -> Integrator/1
  Mux/1 -> Interpreted MATLAB Function/1
  Integrator/1 -> Mux/3, Xp/1

== system battery_cell_model/Pade Approximation Battery Cell Model with Degradation/Pade Approximation Battery Cell Model with Degradation/Negative Electrode/Dynamics ==
  Time : Inport
  Current : Inport  Port=2
  Integrator : Integrator  InitialCondition=x_initial_n_pade_D
  Interpreted MATLAB Function : MATLABFcn  MATLABFcn=state_eqns_pade_d_n
  Mux : Mux  Inputs=3
  C_n : Outport
  wires:
  Current/1 -> Mux/2
  Time/1 -> Mux/1
  Mux/1 -> Interpreted MATLAB Function/1
  Interpreted MATLAB Function/1 -> Integrator/1
  Integrator/1 -> C_n/1, Mux/3

== system battery_cell_model/Pade Approximation Battery Cell Model with Degradation/Pade Approximation Battery Cell Model with Degradation/Negative Electrode/Output C ==
  Time : Inport
  Current : Inport  Port=2
  C_n : Inport  Port=3
  Interpreted MATLAB Function1 : MATLABFcn  MATLABFcn=output_C_pade_D_n
  Mux : Mux  Inputs=3
  Cs,n : Outport
  wires:
  Time/1 -> Mux/1
  Mux/1 -> Interpreted MATLAB Function1/1
  Interpreted MATLAB Function1/1 -> Cs,n/1
  C_n/1 -> Mux/3
  Current/1 -> Mux/2

== system battery_cell_model/Pade Approximation Battery Cell Model with Degradation/Pade Approximation Battery Cell Model with Degradation/Negative Electrode/Side reaction current density ==
  Time : Inport
  Current : Inport  Port=2
  Cs,n : Inport  Port=3
  Interpreted MATLAB Function : MATLABFcn  MATLABFcn=side_reaction
  Mux : Mux  Inputs=3
  J_s : Outport
  wires:
  Interpreted MATLAB Function/1 -> J_s/1
  Time/1 -> Mux/1
  Current/1 -> Mux/2
  Mux/1 -> Interpreted MATLAB Function/1
  Cs,n/1 -> Mux/3

== system battery_cell_model/Pade Approximation Battery Cell Model with Degradation/Pade Approximation Battery Cell Model with Degradation/Positive Electrode/Dynamics ==
  Time : Inport
  Current : Inport  Port=2
  Integrator : Integrator  InitialCondition=x_initial_p_pade_D
  Interpreted MATLAB Function : MATLABFcn  MATLABFcn=state_eqns_pade_d_p
  Mux : Mux  Inputs=3
  C_p : Outport
  wires:
  Current/1 -> Mux/2
  Time/1 -> Mux/1
  Interpreted MATLAB Function/1 -> Integrator/1
  Mux/1 -> Interpreted MATLAB Function/1
  Integrator/1 -> C_p/1, Mux/3

== system battery_cell_model/Pade Approximation Battery Cell Model with Degradation/Pade Approximation Battery Cell Model with Degradation/Positive Electrode/Output C ==
  Time : Inport
  C_p : Inport  Port=2
  Interpreted MATLAB Function1 : MATLABFcn  MATLABFcn=output_C_pade_D_p
  Mux : Mux  Inputs=2
  Cs,p : Outport
  wires:
  Time/1 -> Mux/1
  Mux/1 -> Interpreted MATLAB Function1/1
  Interpreted MATLAB Function1/1 -> Cs,p/1
  C_p/1 -> Mux/2

== system battery_cell_model/Pade Apprximation Battery Cell Model/Pade Apprximation Battery Cell Model/Negative Electrode/Dynamics ==
  Time : Inport
  Current : Inport  Port=2
  Integrator : Integrator  InitialCondition=x_initial_n_pade
  Interpreted MATLAB Function : MATLABFcn  MATLABFcn=state_eqns_pade_n
  Mux : Mux  Inputs=3
  C_n : Outport
  wires:
  Current/1 -> Mux/2
  Time/1 -> Mux/1
  Interpreted MATLAB Function/1 -> Integrator/1
  Mux/1 -> Interpreted MATLAB Function/1
  Integrator/1 -> Mux/3, C_n/1

== system battery_cell_model/Pade Apprximation Battery Cell Model/Pade Apprximation Battery Cell Model/Negative Electrode/Output C ==
  Time : Inport
  C_n : Inport  Port=2
  Interpreted MATLAB Function1 : MATLABFcn  MATLABFcn=output_C_pade_n
  Mux : Mux  Inputs=2
  Cs,n : Outport
  wires:
  Time/1 -> Mux/1
  Mux/1 -> Interpreted MATLAB Function1/1
  Interpreted MATLAB Function1/1 -> Cs,n/1
  C_n/1 -> Mux/2

== system battery_cell_model/Pade Apprximation Battery Cell Model/Pade Apprximation Battery Cell Model/Positive Electrode/Dynamics ==
  Time : Inport
  Current : Inport  Port=2
  Integrator : Integrator  InitialCondition=x_initial_p_pade
  Interpreted MATLAB Function : MATLABFcn  MATLABFcn=state_eqns_pade_p
  Mux : Mux  Inputs=3
  C_p : Outport
  wires:
  Current/1 -> Mux/2
  Time/1 -> Mux/1
  Interpreted MATLAB Function/1 -> Integrator/1
  Mux/1 -> Interpreted MATLAB Function/1
  Integrator/1 -> Mux/3, C_p/1

== system battery_cell_model/Pade Apprximation Battery Cell Model/Pade Apprximation Battery Cell Model/Positive Electrode/Output C ==
  Time : Inport
  C_p : Inport  Port=2
  Interpreted MATLAB Function1 : MATLABFcn  MATLABFcn=output_C_pade_p
  Mux : Mux  Inputs=2
  Cs,p : Outport
  wires:
  Time/1 -> Mux/1
  Mux/1 -> Interpreted MATLAB Function1/1
  Interpreted MATLAB Function1/1 -> Cs,p/1
  C_p/1 -> Mux/2
